simulink model "Assignment_2_3K04"  (R2020a)
settings: Solver=FixedStepAuto  StartTime=0.0  StopTime=1  FixedStep=1e-3  RelTol=1e-3  EnableMultiTasking=on
undefined symbols (not defined in the file): A0, A1, D0, D1, D10, D11, D12, D13, D2, D3, D4, D5, D6, D7, D8, D9, PTA0, PTA1, PTA2, PTB2, PTB23, PTB3, PTB9, PTC16, PTC17, PTC2, PTC3, PTC4, PTD0, PTD1, PTD2, PTD3
libraries: frdmk64flib x20, etargetslib x6, dspstat3 x1
settings Model: ExtModeTrigDuration=5  Creator=Stephen Oh  LastModifiedBy=Ahmed Nazir
settings OptimizationCC: EnhancedBackFolding=on  PassReuseOutputArgsAs=Individual arguments  ZeroExternalMemoryAtStartup=off  ZeroInternalMemoryAtStartup=off  MaxStackSize=64  OptimizeBlockOrder=speed  DifferentSizesBufferReuse=on  OptimizationCustomize=off  EfficientTunableParamExpr=on
settings DebuggingCC: ParameterTunabilityLossMsg=error
settings HardwareCC: ProdBitPerPointer=32  ProdBitPerSizeT=32  ProdBitPerPtrDiffT=32  ProdLargestAtomicInteger=Long  ProdLargestAtomicFloat=Double  ProdWordSize=32  ProdHWDeviceType=ARM Compatible->ARM Cortex
settings SFSimCC: MATLABDynamicMemAlloc=off
settings RTWCC: SystemTargetFile=ert.tlc  HardwareBoard=NXP FRDM-K64F  TemplateMakefile=ert_default_tmf  Toolchain=GNU Tools for ARM Embedded Processors
settings CodeAppCC: ForceParamTrailComments=on  IgnoreCustomStorageClasses=off  OperatorAnnotations=on  SimulinkDataObjDesc=on  SFDataObjDesc=on  InsertBlockDesc=on

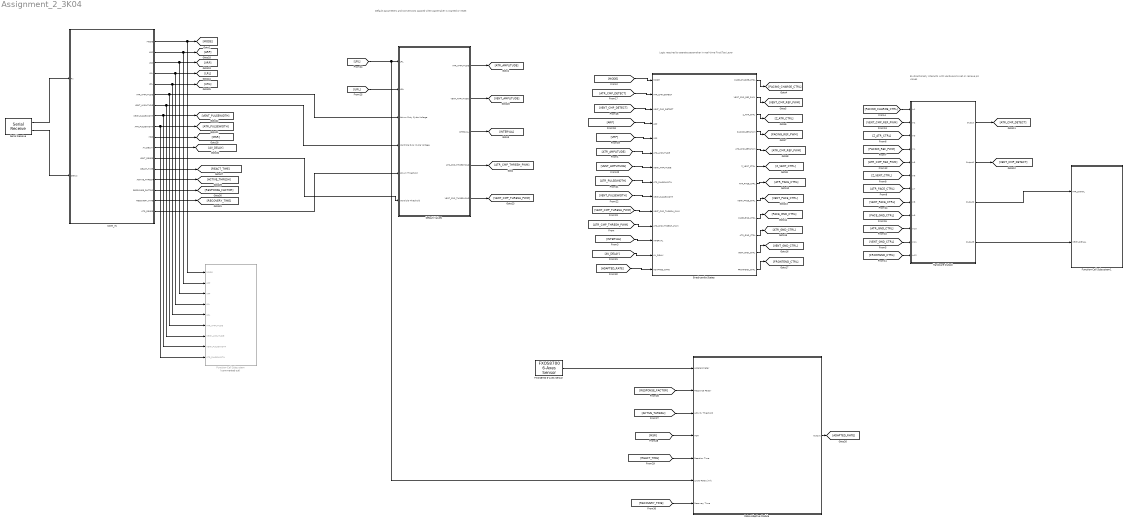
== system Assignment_2_3K04 ==
  note: Default parameters and Conversions passed when
      | pacemaker is started or reset
  note: Logic required to operate pacemaker
      | in real-time
      | First/Top Layer
  note: Bi-directionally interacts with
      | Hardware to set or recieve
      | pin values
  Bradycardia States : Stateflow chart  TreatAsAtomicUnit=on
      settings: PortSchema="{\"entries\":[{\"content\":{\"sides\":[{\"content\":{\"connectorIds\":[\"In2\",\"In3\",\"In4\",\"In5\",\"In6\",\"In7\",\"In8\",\"In9\",\"In10\",\"In11\",\"In12\",\"In1\",\"In13\",\"In14\"]},\"type\":\"ConnectorPlacement.EquallySpacedRectSide\",\"uuid\":\"15e03f69-5c25-4f3e-b3fb-d71978e552f4\"},{\"content\":{\"connectorIds\":[\"Out7\",\"Out12\",\"Out4\",\"Out8\",\"Out10\",\"Out5\",\"Out9\",\"Out3\",\"Out6\",\"Out1\",\"Out2\",\"Out11\"],\"side\":\"RIGHT\"},\"type\":\"ConnectorPlacement.EquallySpacedRectSide\",\"uuid\":\"02171bf1-edb1-4b01-9e56-a8642c556ed6\"},{\"content\":{\"connectorIds\":[],\"side\":\"TOP\"},\"type\":\"ConnectorPlacement.EquallySpacedRectSide\",\"uuid\":\"cc6b5506-3435-4740-9e3f-4dfe15d30bff\"}]},\"type\":\"ConnectorPlacement.EquallySpacedConnector\",\"uuid\":\"0ad55da7-1e65-48d0-a0a4-2620ffa94320\"}],\"packageUris\":[\"http://schema.mathworks.com/mf0/Connector/19700101\"],\"version\":\"1.0\"}"
  COM_IN : Stateflow chart  TreatAsAtomicUnit=on
      settings: PortSchema="{\"entries\":[{\"content\":{\"sides\":[{\"content\":{\"connectorIds\":[\"In1\",\"In2\"]},\"type\":\"ConnectorPlacement.EquallySpacedRectSide\",\"uuid\":\"22fa9edc-2a49-4280-8e8e-0842a45ddb47\"},{\"content\":{\"connectorIds\":[\"Out1\",\"Out2\",\"Out5\",\"Out3\",\"Out4\",\"Out6\",\"Out7\",\"Out8\",\"Out9\",\"Out10\",\"Out11\",\"Out12\",\"Out13\",\"Out14\",\"Out15\",\"Out16\",\"Out17\"],\"side\":\"RIGHT\"},\"type\":\"ConnectorPlacement.EquallySpacedRectSide\",\"uuid\":\"653d204d-01e6-4b1d-8e7b-47ebaddcd032\"},{\"content\":{\"connectorIds\":[],\"side\":\"TOP\"},\"type\":\"ConnectorPlacement.EquallySpacedRectSide\",\"uuid\":\"5fb759fd-937e-492d-8a65-272e5a7048d8\"}]},\"type\":\"ConnectorPlacement.EquallySpacedConnector\",\"uuid\":\"8ef65fa3-58c0-4e1e-983b-59a6af0cca9a\"}],\"packageUris\":[\"http://schema.mathworks.com/mf0/Connector/19700101\"],\"version\":\"1.0\"}"
  Default Values : Subsystem
  FXOS8700 6-Axes Sensor : frdmk64flib/FXOS8700 6-Axes Sensor  Activesensor=Accelerometer only  ODR=800Hz  HybridODR=400Hz  Accelfullrange=-4g to +4g  SampleTime=-1
  Function-Call Subsystem : Subsystem  Commented=on  TreatAsAtomicUnit=on
  Function-Call Subsystem1 : Subsystem  TreatAsAtomicUnit=on
  Hardware Output : Subsystem
  Rate Adaptive Module : Subsystem
  Serial Receive : frdmk64flib/Serial Receive  SCIModule=0  Baudrate=uint32(9600)  Parity=None  StopBits=1  HardwareFlowControl=None  ByteOrder=LittleEndian  DataType=uint8  DataLength=37  BlockingMode=off  OutputStatus=on  SampleTime=-1
  wires:
  [INTERVAL] -> Bradycardia States/1(INTERVAL)
  [ATR_GND_CTRL] -> Hardware Output/10(In10)
  [PACING_REF_PWM] -> Hardware Output/4(In4)
  [Z_VENT_CTRL] -> Hardware Output/6(In6)
  [ATR_PACE_CTRL] -> Hardware Output/7(In7)
  Hardware Output/2(Output1) -> [VENT_CMP_DETECT]
  [PACE_GND_CTRL] -> Hardware Output/9(In9)
  [FRONTEND_CTRL] -> Hardware Output/12(In12)
  [VENT_GND_CTRL] -> Hardware Output/11(In11)
  [Z_ATR_CTRL] -> Hardware Output/3(In3)
  [VENT_PACE_CTRL] -> Hardware Output/8(In8)
  [ATR_CMP_REF_PWM] -> Hardware Output/5(In5)
  [VENT_CMP_REF_PWM] -> Hardware Output/2(In2)
  [PACING_CHARGE_CTRL] -> Hardware Output/1(In1)
  Hardware Output/1(Output) -> [ATR_CMP_DETECT]
  [VENT_CMP_DETECT] -> Bradycardia States/4(VENT_CMP_DETECT)
  [ARP] -> Bradycardia States/5(ARP)
  [VRP] -> Bradycardia States/6(VRP)
  [ATR_CMP_DETECT] -> Bradycardia States/3(ATR_CMP_DETECT)
  [ATR_AMPLITUDE] -> Bradycardia States/7(ATR_AMPLITUDE)
  [VENT_AMPLITUDE] -> Bradycardia States/8(VENT_AMPLITUDE)
  [ATR_PULSEWIDTH] -> Bradycardia States/9(ATR_PULSEWIDTH)
  [VENT_PULSEWIDTH] -> Bradycardia States/10(VENT_PULSEWIDTH)
  Default Values/1(ATR_AMPLITUDE) -> [ATR_AMPLITUDE]
  Default Values/3(INTERVAL) -> [INTERVAL]
  Bradycardia States/3(VENT_PACE_CTRL) -> [VENT_PACE_CTRL]
  Bradycardia States/9(ATR_PACE_CTRL) -> [ATR_PACE_CTRL]
  Bradycardia States/7(PACE_CHARGE_CTRL) -> [PACING_CHARGE_CTRL]
  Bradycardia States/12(VENT_CMP_REF_PWM) -> [VENT_CMP_REF_PWM]
  Bradycardia States/4(Z_ATR_CTRL) -> [Z_ATR_CTRL]
  Bradycardia States/8(PACING_REF_PWM) -> [PACING_REF_PWM]
  Bradycardia States/10(ATR_CMP_REF_PWM) -> [ATR_CMP_REF_PWM]
  Bradycardia States/5(Z_VENT_CTRL) -> [Z_VENT_CTRL]
  Bradycardia States/6(PACE_GND_CTRL) -> [PACE_GND_CTRL]
  Bradycardia States/1(ATR_GND_CTRL) -> [ATR_GND_CTRL]
  Bradycardia States/2(VENT_GND_CTRL) -> [VENT_GND_CTRL]
  Bradycardia States/11(FRONTEND_CTRL) -> [FRONTEND_CTRL]
  [ATR_CMP_THRESH_PWM] -> Bradycardia States/12(ATR_CMP_THRESH_PWM)
  [VENT_CMP_THRESH_PWM] -> Bradycardia States/11(VENT_CMP_THRESH_PWM)
  Serial Receive/1 -> COM_IN/1(Rx)
  Serial Receive/2 -> COM_IN/2(Status)
  COM_IN/1(MODE) -> Function-Call Subsystem/1(MODE), [MODE]
  [MODE] -> Bradycardia States/2(MODE)
  COM_IN/2(ARP) -> Function-Call Subsystem/2(ARP), [ARP]
  COM_IN/5(VRP) -> Function-Call Subsystem/3(VRP), [VRP]
  COM_IN/6(ATR_AMPLITUDE) -> Function-Call Subsystem/6(ATR_AMPLITUDE), Default Values/3(Atrium Duty Cycle Voltage)
  COM_IN/7(VENT_AMPLITUDE) -> Function-Call Subsystem/7(VENT_AMPLITUDE), Default Values/4(Ventricle Duty Cycle Voltage)
  Default Values/2(VENT_AMPLITUDE) -> [VENT_AMPLITUDE]
  COM_IN/3(LRL) -> Function-Call Subsystem/4(LRL), [LRL]
  COM_IN/4(URL) -> Function-Call Subsystem/5(URL), [URL]
  [URL] -> Default Values/2(URL)
  COM_IN/13(REACT_TIME) -> [REACT_TIME]
  COM_IN/10(MSR) -> [MSR]
  COM_IN/14(ACTIVE_THRESH) -> [ACTIVE_THRESH]
  COM_IN/15(RESPONSE_FACTOR) -> [RESPONSE_FACTOR]
  COM_IN/16(RECOVERY_TIME) -> [RECOVERY_TIME]
  COM_IN/11(AV_DELAY) -> [AV_DELAY]
  [AV_DELAY] -> Bradycardia States/13(AV_DELAY)
  [ADAPTED_RATE] -> Bradycardia States/14(ADAPTED_RATE)
  COM_IN/8(VENT_PULSEWIDTH) -> Function-Call Subsystem/8(VENT_PULSEWIDTH), [VENT_PULSEWIDTH]
  COM_IN/9(ATR_PULSEWIDTH) -> Function-Call Subsystem/9(ATR_PULSEWIDTH), [ATR_PULSEWIDTH]
  Default Values/4(ATR_CMP_THRESHOLD) -> [ATR_CMP_THRESH_PWM]
  Default Values/5(VENT_CMP_THRESHOLD) -> [VENT_CMP_THRESH_PWM]
  COM_IN/12(VENT_SENSE) -> Default Values/6(Ventricle Threshold)
  COM_IN/17(ATR_SENSE) -> Default Values/5(Atrium Threshold)
  FXOS8700 6-Axes Sensor/1 -> Rate Adaptive Module/1(Accelerometer)
  Rate Adaptive Module/1(Output) -> [ADAPTED_RATE]
  [RESPONSE_FACTOR] -> Rate Adaptive Module/2(Response Factor)
  [ACTIVE_THRESH] -> Rate Adaptive Module/3(Activity Threshold)
  [MSR] -> Rate Adaptive Module/4(MSR)
  [REACT_TIME] -> Rate Adaptive Module/5(Reaction Time)
  [LRL] -> Rate Adaptive Module/6(Lower Rate Limit), Default Values/1(LRL)
  [RECOVERY_TIME] -> Rate Adaptive Module/7(Recovery Time)
  Hardware Output/3(Output2) -> Function-Call Subsystem1/1(ATR_SIGNAL)
  Hardware Output/4(Output3) -> Function-Call Subsystem1/2(VENT_SIGNAL)

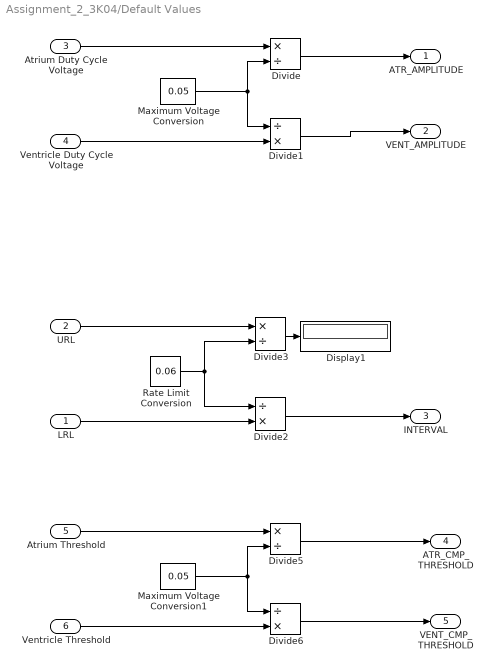
== system Assignment_2_3K04/Default Values ==
  LRL : Inport
  URL : Inport  Port=2
  Atrium Duty Cycle Voltage : Inport  Port=3  OutDataTypeStr=single
  Ventricle Duty Cycle Voltage : Inport  Port=4  OutDataTypeStr=single
  Atrium Threshold : Inport  Port=5  OutDataTypeStr=single
  Ventricle Threshold : Inport  Port=6  OutDataTypeStr=single
  Display1 : Display
  Divide : Product  Inputs=*/  OutDataTypeStr=uint8
  Divide1 : Product  Inputs=/*  OutDataTypeStr=uint8
  Divide2 : Product  Inputs=/*
  Divide3 : Product  Inputs=*/
  Divide5 : Product  Inputs=*/  OutDataTypeStr=uint8
  Divide6 : Product  Inputs=/*  OutDataTypeStr=uint8
  Maximum Voltage Conversion : Constant  Value=0.05
  Maximum Voltage Conversion1 : Constant  Value=0.05
  Rate Limit Conversion : Constant  Value=0.06
  ATR_AMPLITUDE : Outport  OutDataTypeStr=uint8
  VENT_AMPLITUDE : Outport  Port=2  OutDataTypeStr=uint8
  INTERVAL : Outport  Port=3
  ATR_CMP_THRESHOLD : Outport  Port=4  OutDataTypeStr=uint8
  VENT_CMP_THRESHOLD : Outport  Port=5  OutDataTypeStr=uint8
  wires:
  Divide2/1 -> INTERVAL/1
  Maximum Voltage Conversion/1 -> Divide1/1, Divide/2
  Rate Limit Conversion/1 -> Divide3/2, Divide2/1
  URL/1 -> Divide3/1
  Divide3/1 -> Display1/1
  Atrium Duty Cycle Voltage/1 -> Divide/1
  Ventricle Duty Cycle Voltage/1 -> Divide1/2
  Divide/1 -> ATR_AMPLITUDE/1
  Divide1/1 -> VENT_AMPLITUDE/1
  Divide6/1 -> VENT_CMP_THRESHOLD/1
  Maximum Voltage Conversion1/1 -> Divide6/1, Divide5/2
  Atrium Threshold/1 -> Divide5/1
  Divide5/1 -> ATR_CMP_THRESHOLD/1
  Ventricle Threshold/1 -> Divide6/2
  LRL/1 -> Divide2/2

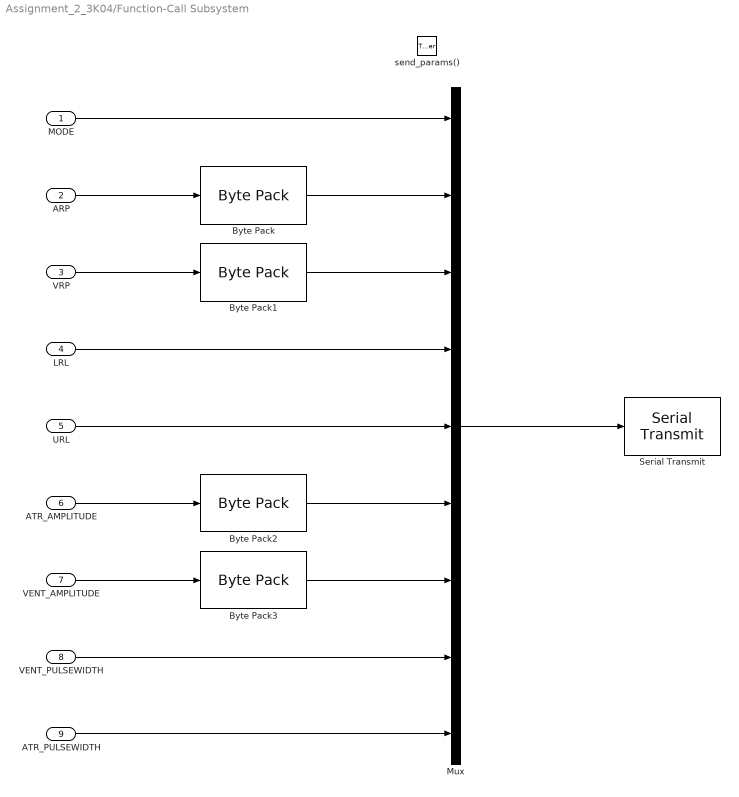
== system Assignment_2_3K04/Function-Call Subsystem ==
  MODE : Inport  OutDataTypeStr=uint8
  ARP : Inport  Port=2
  VRP : Inport  Port=3
  LRL : Inport  Port=4
  URL : Inport  Port=5
  ATR_AMPLITUDE : Inport  Port=6
  VENT_AMPLITUDE : Inport  Port=7
  VENT_PULSEWIDTH : Inport  Port=8
  ATR_PULSEWIDTH : Inport  Port=9
  send_params() : TriggerPort  TriggerType=function-call  IsSimulinkFunction=on  FunctionName=send_params  VariantControl=Variant
  Byte Pack : etargetslib/Byte Pack  datatypes={'uint16'}  byteAlign=1
  Byte Pack1 : etargetslib/Byte Pack  datatypes={'uint16'}  byteAlign=1
  Byte Pack2 : etargetslib/Byte Pack  datatypes={'single'}  byteAlign=1
  Byte Pack3 : etargetslib/Byte Pack  datatypes={'single'}  byteAlign=1
  Mux : Mux  Inputs=9
  Serial Transmit : frdmk64flib/Serial Transmit  SCIModule=0  Baudrate=uint32(9600)  Parity=None  StopBits=1  HardwareFlowControl=None  ByteOrder=LittleEndian  BlockingMode=on  OutputStatus=off
  wires:
  Mux/1 -> Serial Transmit/1
  ARP/1 -> Byte Pack/1
  VRP/1 -> Byte Pack1/1
  LRL/1 -> Mux/4
  URL/1 -> Mux/5
  ATR_AMPLITUDE/1 -> Byte Pack2/1
  VENT_AMPLITUDE/1 -> Byte Pack3/1
  VENT_PULSEWIDTH/1 -> Mux/8
  ATR_PULSEWIDTH/1 -> Mux/9
  MODE/1 -> Mux/1
  Byte Pack/1 -> Mux/2
  Byte Pack1/1 -> Mux/3
  Byte Pack2/1 -> Mux/6
  Byte Pack3/1 -> Mux/7

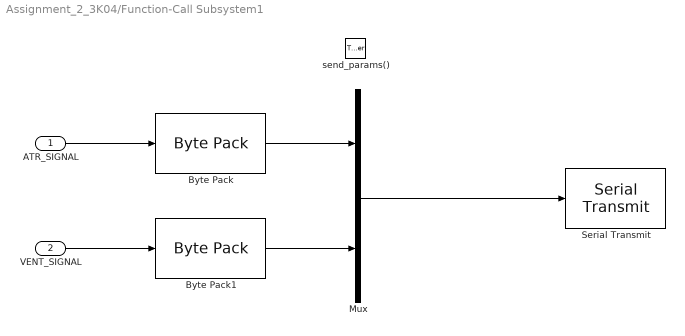
== system Assignment_2_3K04/Function-Call Subsystem1 ==
  ATR_SIGNAL : Inport  OutDataTypeStr=double
  VENT_SIGNAL : Inport  Port=2  OutDataTypeStr=double
  send_params() : TriggerPort  TriggerType=function-call  IsSimulinkFunction=on  FunctionName=send_params  VariantControl=Variant
  Byte Pack : etargetslib/Byte Pack  datatypes={'double'}  byteAlign=1
  Byte Pack1 : etargetslib/Byte Pack  datatypes={'double'}  byteAlign=1
  Mux : Mux  Inputs=2
  Serial Transmit : frdmk64flib/Serial Transmit  SCIModule=0  Baudrate=uint32(9600)  Parity=None  StopBits=1  HardwareFlowControl=None  ByteOrder=LittleEndian  BlockingMode=on  OutputStatus=off
  wires:
  ATR_SIGNAL/1 -> Byte Pack/1
  Mux/1 -> Serial Transmit/1
  VENT_SIGNAL/1 -> Byte Pack1/1
  Byte Pack/1 -> Mux/1
  Byte Pack1/1 -> Mux/2

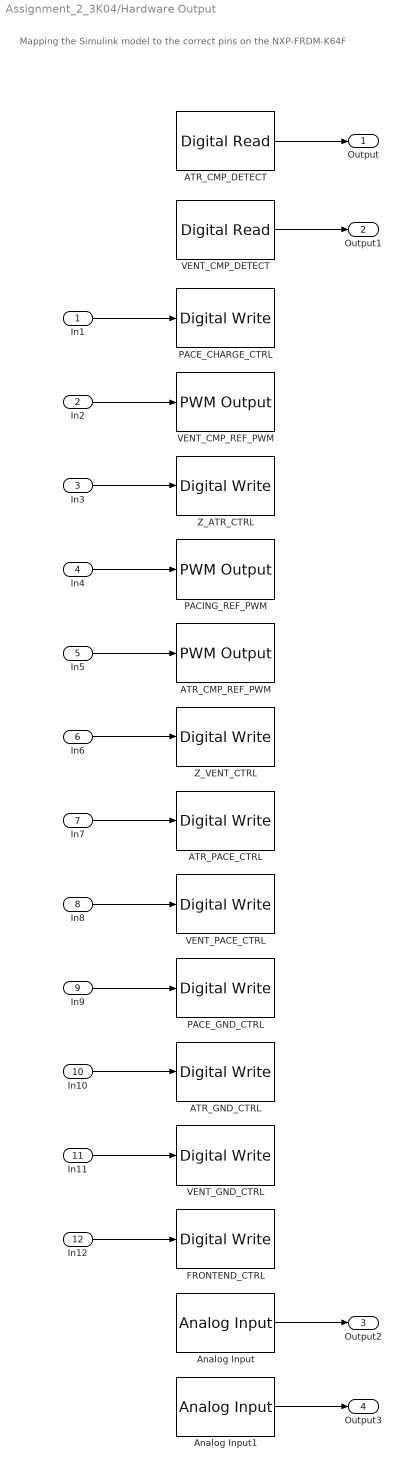
== system Assignment_2_3K04/Hardware Output ==
  note: Mapping the Simulink model to the correct pins
      | on the NXP-FRDM-K64F
  In1 : Inport
  In2 : Inport  Port=2
  In3 : Inport  Port=3
  In4 : Inport  Port=4
  In5 : Inport  Port=5
  In6 : Inport  Port=6
  In7 : Inport  Port=7
  In8 : Inport  Port=8
  In9 : Inport  Port=9
  In10 : Inport  Port=10
  In11 : Inport  Port=11
  In12 : Inport  Port=12
  ATR_CMP_DETECT : frdmk64flib/Digital Read  Whichpin=PTC16 (D0)  SampleTime=-1
  ATR_CMP_REF_PWM : frdmk64flib/PWM Output  Whichpin=PTC2 (D6)  InitialFrequency=2000  InitialDutyCycle=30
  ATR_GND_CTRL : frdmk64flib/Digital Write  Whichpin=PTD2 (D11)
  ATR_PACE_CTRL : frdmk64flib/Digital Write  Whichpin=PTA0 (D8)
  Analog Input : frdmk64flib/Analog Input  Whichpin=PTB2 (A0)  SampleTime=-1
  Analog Input1 : frdmk64flib/Analog Input  Whichpin=PTB3 (A1)  SampleTime=-1
  FRONTEND_CTRL : frdmk64flib/Digital Write  Whichpin=PTD1 (D13)
  PACE_CHARGE_CTRL : frdmk64flib/Digital Write  Whichpin=PTB9 (D2)
  PACE_GND_CTRL : frdmk64flib/Digital Write  Whichpin=PTD0 (D10)
  PACING_REF_PWM : frdmk64flib/PWM Output  Whichpin=PTA2 (D5)  InitialFrequency=2000  InitialDutyCycle=30
  VENT_CMP_DETECT : frdmk64flib/Digital Read  Whichpin=PTC17 (D1)  SampleTime=-1
  VENT_CMP_REF_PWM : frdmk64flib/PWM Output  Whichpin=PTA1 (D3)  InitialFrequency=2000  InitialDutyCycle=30
  VENT_GND_CTRL : frdmk64flib/Digital Write  Whichpin=PTD3 (D12)
  VENT_PACE_CTRL : frdmk64flib/Digital Write  Whichpin=PTC4 (D9)
  Z_ATR_CTRL : frdmk64flib/Digital Write  Whichpin=PTB23 (D4)
  Z_VENT_CTRL : frdmk64flib/Digital Write  Whichpin=PTC3 (D7)
  Output : Outport
  Output1 : Outport  Port=2
  Output2 : Outport  Port=3  OutDataTypeStr=double
  Output3 : Outport  Port=4  OutDataTypeStr=double
  wires:
  In1/1 -> PACE_CHARGE_CTRL/1
  ATR_CMP_DETECT/1 -> Output/1
  VENT_CMP_DETECT/1 -> Output1/1
  In2/1 -> VENT_CMP_REF_PWM/1
  In3/1 -> Z_ATR_CTRL/1
  In4/1 -> PACING_REF_PWM/1
  In5/1 -> ATR_CMP_REF_PWM/1
  In6/1 -> Z_VENT_CTRL/1
  In7/1 -> ATR_PACE_CTRL/1
  In8/1 -> VENT_PACE_CTRL/1
  In9/1 -> PACE_GND_CTRL/1
  In10/1 -> ATR_GND_CTRL/1
  In11/1 -> VENT_GND_CTRL/1
  In12/1 -> FRONTEND_CTRL/1
  Analog Input/1 -> Output2/1
  Analog Input1/1 -> Output3/1

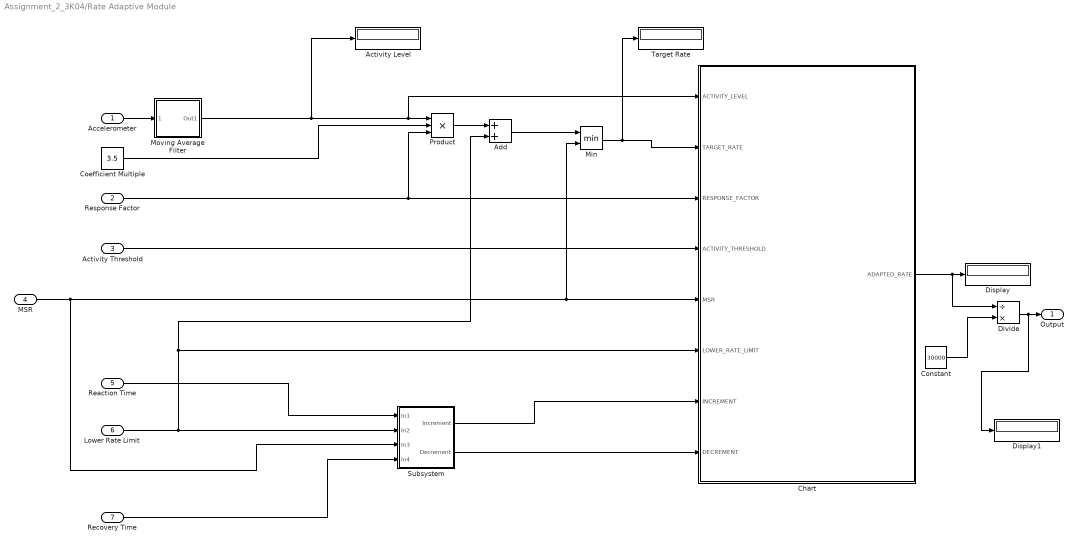
== system Assignment_2_3K04/Rate Adaptive Module ==
  Accelerometer : Inport
  Response Factor : Inport  Port=2
  Activity Threshold : Inport  Port=3
  MSR : Inport  Port=4
  Reaction Time : Inport  Port=5
  Lower Rate Limit : Inport  Port=6
  Recovery Time : Inport  Port=7
  Activity Level : Display
  Add : Sum
  Chart : Stateflow chart  TreatAsAtomicUnit=on
      settings: PortSchema="{\"entries\":[{\"content\":{\"sides\":[{\"content\":{\"connectorIds\":[\"In1\",\"In3\",\"In2\",\"In6\",\"In8\",\"In7\",\"In4\",\"In5\"]},\"type\":\"ConnectorPlacement.EquallySpacedRectSide\",\"uuid\":\"efebee7e-2c09-4b25-ba04-904f72c011ed\"},{\"content\":{\"connectorIds\":[\"Out1\"],\"side\":\"RIGHT\"},\"type\":\"ConnectorPlacement.EquallySpacedRectSide\",\"uuid\":\"6322cc63-1b7a-423a-b49b-7b27e71e0c32\"},{\"content\":{\"connectorIds\":[],\"side\":\"TOP\"},\"type\":\"ConnectorPlacement.EquallySpacedRectSide\",\"uuid\":\"daf2dbd4-7676-46e9-bb01-958bd0e2e14e\"}]},\"type\":\"ConnectorPlacement.EquallySpacedConnector\",\"uuid\":\"43c3c7b3-b94c-45f5-b310-1a430cfb2b71\"}],\"packageUris\":[\"http://schema.mathworks.com/mf0/Connector/19700101\"],\"version\":\"1.0\"}"
  Coefficient Multiple : Constant  Value=3.5
  Constant : Constant  Value=30000
  Display : Display
  Display1 : Display
  Divide : Product  Inputs=/*
  Min : MinMax  Inputs=2
  Moving Average Filter : Subsystem
  Product : Product  Inputs=3
  Subsystem : Subsystem
  Target Rate : Display
  Output : Outport
  wires:
  Recovery Time/1 -> Subsystem/4(In4)
  MSR/1 -> Subsystem/3(In3), Min/2, Chart/8(MSR)
  Subsystem/1(Increment) -> Chart/4(INCREMENT)
  Activity Threshold/1 -> Chart/6(ACTIVITY_THRESHOLD)
  Response Factor/1 -> Product/3, Chart/2(RESPONSE_FACTOR)
  Lower Rate Limit/1 -> Subsystem/2(In2), Chart/7(LOWER_RATE_LIMIT), Add/2
  Add/1 -> Min/1
  Product/1 -> Add/1
  Min/1 -> Target Rate/1, Chart/3(TARGET_RATE)
  Reaction Time/1 -> Subsystem/1(In1)
  Subsystem/2(Decrement) -> Chart/5(DECREMENT)
  Chart/1(ADAPTED_RATE) -> Divide/1, Display/1
  Coefficient Multiple/1 -> Product/2
  Divide/1 -> Display1/1, Output/1
  Constant/1 -> Divide/2
  Moving Average Filter/1(Out1) -> Activity Level/1, Chart/1(ACTIVITY_LEVEL), Product/1
  Accelerometer/1 -> Moving Average Filter/1(Accelerometer)

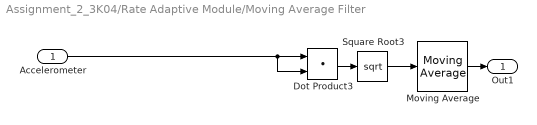
== system Assignment_2_3K04/Rate Adaptive Module/Moving Average Filter ==
  Accelerometer : Inport
  Dot Product3 : DotProduct  InputSameDT=on  OutDataTypeStr=Inherit: Inherit via internal rule
  Moving Average : dspstat3/Moving Average  Method=Sliding window  ForgettingFactorPort=off  SpecifyWindowLength=on  WindowLength=500  ForgettingFactor=0.9  SimulateUsing=Code generation
  Square Root3 : Sqrt  SaturateOnIntegerOverflow=on
  Out1 : Outport
  wires:
  Accelerometer/1 -> Dot Product3/2, Dot Product3/1
  Dot Product3/1 -> Square Root3/1
  Square Root3/1 -> Moving Average/1
  Moving Average/1 -> Out1/1

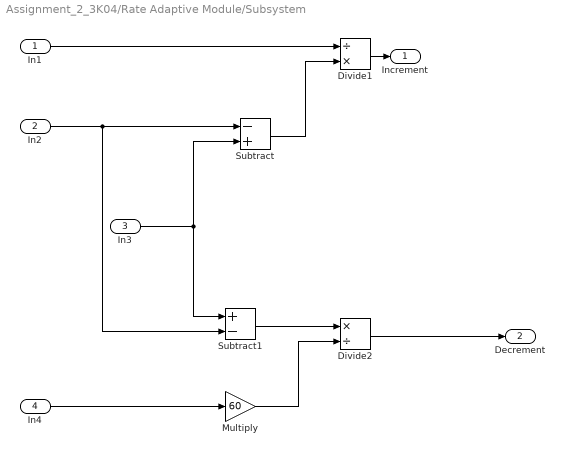
== system Assignment_2_3K04/Rate Adaptive Module/Subsystem ==
  In1 : Inport
  In2 : Inport  Port=2
  In3 : Inport  Port=3
  In4 : Inport  Port=4
  Divide1 : Product  Inputs=/*  OutDataTypeStr=uint8  RndMeth=Ceiling
  Divide2 : Product  Inputs=*/  OutDataTypeStr=uint8  RndMeth=Ceiling  SaturateOnIntegerOverflow=on
  Multiply : Gain  Gain=60
  Subtract : Sum  Inputs=-+
  Subtract1 : Sum  Inputs=+-
  Increment : Outport
  Decrement : Outport  Port=2
  wires:
  Multiply/1 -> Divide2/2
  In2/1 -> Subtract1/2, Subtract/1
  In3/1 -> Subtract/2, Subtract1/1
  Divide1/1 -> Increment/1
  In1/1 -> Divide1/1
  Subtract1/1 -> Divide2/1
  Subtract/1 -> Divide1/2
  In4/1 -> Multiply/1
  Divide2/1 -> Decrement/1

== stateflow chart Assignment_2_3K04/COM_IN ==
  state SET_PARAM
    entry:
    MODE = Rx(3);
    LRL = Rx(4);
    URL = Rx(5);
    ATR_AMPLITUDE = typecast(Rx(6:9),'single');
    VENT_AMPLITUDE = typecast(Rx(10:13),'single');
    ATR_PULSEWIDTH = Rx(14);
    VENT_PULSEWIDTH = Rx(15);
    ARP = typecast(Rx(16:17),'uint16');
    VRP = typecast(Rx(18:19),'uint16');
    ATR_SENSE = typecast(Rx(20:23),'single');
    VENT_SENSE = typecast(Rx(24:27),'single');
    MSR = Rx(28);
    RECOVERY_TIME = Rx(29);
    REACT_TIME = Rx(30);
    RESPONSE_FACTOR = Rx(31);
    ACTIVE_THRESH = typecast(Rx(32:35),'single');
    AV_DELAY = typecast(Rx(36:37),'uint16');
    %Get the values from DCM
  state INITIAL
    %Set all Nomial Values
    entry:
    MODE = 5;
    LRL = 60;
    URL = 120;
    ATR_AMPLITUDE = 5;
    VENT_AMPLITUDE = 5;
    ATR_PULSEWIDTH = 2;
    VENT_PULSEWIDTH = 2;
    ARP = 250;
    VRP = 250;
    ATR_SENSE = 4;
    VENT_SENSE = 4;
    MSR = 100;
    RECOVERY_TIME = 2;
    REACT_TIME = 10;
    RESPONSE_FACTOR = 16;
    ACTIVE_THRESH = 1.1;
    AV_DELAY = 100;
  state STANDBY
    %Wait for COM Data
  state ECHO_PARAM
    entry:
    send_params()
  state INITIAL1 [commented out]
    %Set all Nomial Values
    entry:
    MODE = 0;
    LRL = 60;
    URL = 120;
    ATR_AMPLITUDE = 5;
    VENT_AMPLITUDE = 5;
    ATR_PULSEWIDTH = 1;
    VENT_PULSEWIDTH = 1;
    ARP = 250;
    VRP = 320;
    ATR_SENSE = 4;
    VENT_SENSE = 4;
    MSR = 120;
    RECOVERY_TIME = 5;
    REACT_TIME = 30;
    RESPONSE_FACTOR = 8;
    ACTIVE_THRESH = 0;
    AV_DELAY = 150;
  (default) -> INITIAL
  SET_PARAM -> STANDBY
  (junction 13) -> SET_PARAM [order 1] : [Rx(2) == hex2dec('55')]
  (junction 12) -> STANDBY [order 2]
  INITIAL -> STANDBY
  STANDBY -> (junction 12) : [Status==0]
  (junction 12) -> (junction 13) [order 1] : [Rx(1) == hex2dec('16')]
  (junction 13) -> ECHO_PARAM [order 2] : [Rx(2) == hex2dec('22')]
  ECHO_PARAM -> STANDBY
  data: Rx input uint8; Status input uint8; MODE output uint8; ARP output uint16; LRL output uint8; URL output uint8; VRP output uint16; ATR_AMPLITUDE output single; VENT_AMPLITUDE output single; VENT_PULSEWIDTH output uint8; ATR_PULSEWIDTH output uint8; MSR output uint8; AV_DELAY output uint16; VENT_SENSE output single; REACT_TIME output uint8; ACTIVE_THRESH output single; RESPONSE_FACTOR output uint8; RECOVERY_TIME output uint8; ATR_SENSE output single

== stateflow chart Assignment_2_3K04/Rate Adaptive Module/Chart ==
  state RateSelect
    entry:
    ADAPTED_RATE = LOWER_RATE_LIMIT
  state Increment
    entry:
    ADAPTED_RATE = ADAPTED_RATE + INCREMENT
  state TargetRateAchieved
  state Decrement
    entry:
    ADAPTED_RATE = ADAPTED_RATE - DECREMENT
  Increment -> Increment [order 2] : after(1000, msec) [ACTIVITY_LEVEL > ACTIVITY_THRESHOLD]
  (default) -> RateSelect
  Increment -> TargetRateAchieved [order 1] : [ADAPTED_RATE >= TARGET_RATE ]
  RateSelect -> Increment [order 1] : [ACTIVITY_LEVEL > ACTIVITY_THRESHOLD]
  RateSelect -> RateSelect [order 2] : [ACTIVITY_LEVEL < ACTIVITY_THRESHOLD]
  Decrement -> RateSelect [order 3] : [ADAPTED_RATE <= LOWER_RATE_LIMIT]
  Decrement -> Increment [order 1] : after(1000, msec) [ACTIVITY_LEVEL > ACTIVITY_THRESHOLD]
  Increment -> Decrement [order 3] : after(1000, msec) [ACTIVITY_LEVEL < ACTIVITY_THRESHOLD]
  TargetRateAchieved -> Decrement : [ACTIVITY_LEVEL < ACTIVITY_THRESHOLD]
  Decrement -> Decrement [order 2] : after(1000, msec) [ACTIVITY_LEVEL < ACTIVITY_THRESHOLD]
  data: ACTIVITY_LEVEL input; RESPONSE_FACTOR input; ADAPTED_RATE output; TARGET_RATE input; INCREMENT input; DECREMENT input; ACTIVITY_THRESHOLD input; LOWER_RATE_LIMIT input; MSR input

== stateflow chart Assignment_2_3K04/Bradycardia States ==
  note: Second/Structural Layer
  note: Mode Select with Conditional transition to 4 modes
  state ModeSelect
  state AOO [group]
    state Charging
      entry:
      %
      %Charging capacitor C22
      %
      FRONTEND_CTRL = HIGH
      ATR_PACE_CTRL = LOW
      VENT_PACE_CTRL = LOW
      PACING_REF_PWM = ATR_AMPLITUDE
      PACE_CHARGE_CTRL = HIGH
      %
      %Charge release of capacitor C21 into Atrium ground
      %
      PACE_GND_CTRL = HIGH
      VENT_PACE_CTRL = LOW
      Z_ATR_CTRL = LOW
      Z_VENT_CTRL = LOW
      ATR_PACE_CTRL = LOW
      ATR_GND_CTRL = HIGH
      VENT_GND_CTRL = LOW
    state Discharging
      entry:
      %
      %Charge release of capacitor C22 to charge capacitor C21
      %
      PACE_CHARGE_CTRL = LOW
      PACE_GND_CTRL = HIGH
      VENT_PACE_CTRL = LOW
      VENT_GND_CTRL = LOW
      Z_VENT_CTRL = LOW
      Z_ATR_CTRL = LOW
      ATR_GND_CTRL = LOW
      ATR_PACE_CTRL = HIGH
    AOO.Charging -> AOO.Discharging [order 1] : after(delayINTERVAL, msec)
    AOO.Discharging -> AOO.Charging : after(delayATR_PULSEWIDTH, msec)
  state VOO [group]
    state Charging
      entry:
      %
      %Charging capacitor C22
      %
      FRONTEND_CTRL = HIGH
      ATR_PACE_CTRL = LOW
      VENT_PACE_CTRL = LOW
      PACING_REF_PWM = VENT_AMPLITUDE
      PACE_CHARGE_CTRL = HIGH
      %
      %Charge release of capacitor C21 into Ventricle ground
      %
      PACE_GND_CTRL = HIGH
      VENT_PACE_CTRL = LOW
      Z_ATR_CTRL = LOW
      Z_VENT_CTRL = LOW
      ATR_PACE_CTRL = LOW
      ATR_GND_CTRL = LOW
      VENT_GND_CTRL = HIGH
    state Discharging
      entry:
      %
      %Charge release of capacitor C22 to charge capacitor C21
      %
      PACE_CHARGE_CTRL = LOW
      PACE_GND_CTRL = HIGH
      ATR_PACE_CTRL = LOW
      ATR_GND_CTRL = LOW
      Z_VENT_CTRL = LOW
      Z_ATR_CTRL = LOW
      VENT_GND_CTRL = LOW
      VENT_PACE_CTRL = HIGH
    VOO.Charging -> VOO.Discharging [order 1] : after(delayINTERVAL, msec)
    VOO.Discharging -> VOO.Charging : after(delayVENT_PULSEWIDTH, msec)
  state AAI [group]
    state Transition
      %Check for sense outside atrium refractory period
    state Discharging
      entry:
      %Charge release of capacitor C22 to charge capacitor C21
      %
      PACE_CHARGE_CTRL = LOW
      PACE_GND_CTRL = HIGH
      VENT_PACE_CTRL = LOW
      VENT_GND_CTRL = LOW
      Z_VENT_CTRL = LOW
      Z_ATR_CTRL = LOW
      ATR_GND_CTRL = LOW
      ATR_PACE_CTRL = HIGH
    state Charging
      entry:
      %
      %Turn sensing on
      FRONTEND_CTRL = HIGH
      ATR_CMP_REF_PWM = ATR_CMP_THRESH_PWM
      %Charging capacitor C22
      %
      ATR_PACE_CTRL = LOW
      VENT_PACE_CTRL = LOW
      PACING_REF_PWM = ATR_AMPLITUDE
      PACE_CHARGE_CTRL = HIGH
      %Charge release of capacitor C21 into Atrium ground
      PACE_GND_CTRL = HIGH
      VENT_PACE_CTRL = LOW
      Z_ATR_CTRL = LOW
      Z_VENT_CTRL = LOW
      ATR_PACE_CTRL = LOW
      ATR_GND_CTRL = HIGH
      VENT_GND_CTRL = LOW
    AAI.Transition -> AAI.Discharging [order 1] : after(delayINTERVAL-delayARP, msec)
    AAI.Transition -> AAI.Charging [order 2] : [ATR_CMP_DETECT == HIGH]
    AAI.Charging -> AAI.Transition [order 1] : after(delayARP, msec)
    AAI.Discharging -> AAI.Charging : after(delayATR_PULSEWIDTH, msec)
  state VVI [group]
    state Transition
      %Check for sense outside ventricle refractory period
    state Charging
      entry:
      %
      %Turn sensing on
      FRONTEND_CTRL = HIGH
      VENT_CMP_REF_PWM = VENT_CMP_THRESH_PWM
      %Charging capacitor C22
      %
      ATR_PACE_CTRL = LOW
      VENT_PACE_CTRL = LOW
      PACING_REF_PWM = VENT_AMPLITUDE
      PACE_CHARGE_CTRL = HIGH
      %Charge release of capacitor C21 into Ventricle ground
      PACE_GND_CTRL = HIGH
      VENT_PACE_CTRL = LOW
      Z_ATR_CTRL = LOW
      Z_VENT_CTRL = LOW
      ATR_PACE_CTRL = LOW
      ATR_GND_CTRL = LOW
      VENT_GND_CTRL = HIGH
    state Discharging
      entry:
      %Charge release of capacitor C22 to charge capacitor C21
      %
      PACE_CHARGE_CTRL = LOW
      PACE_GND_CTRL = HIGH
      ATR_PACE_CTRL = LOW
      ATR_GND_CTRL = LOW
      Z_VENT_CTRL = LOW
      Z_ATR_CTRL = LOW
      VENT_GND_CTRL = LOW
      VENT_PACE_CTRL = HIGH
    VVI.Transition -> VVI.Discharging [order 1] : after(delayINTERVAL-delayVRP, msec)
    VVI.Transition -> VVI.Charging [order 2] : [VENT_CMP_DETECT == HIGH]
    VVI.Charging -> VVI.Transition [order 1] : after(delayVRP, msec)
    VVI.Discharging -> VVI.Charging : after(delayVENT_PULSEWIDTH, msec)
  state AOOR [group]
    state Charging
      entry:
      %
      %Charging capacitor C22
      %
      FRONTEND_CTRL = HIGH
      ATR_PACE_CTRL = LOW
      VENT_PACE_CTRL = LOW
      PACING_REF_PWM = ATR_AMPLITUDE
      PACE_CHARGE_CTRL = HIGH
      %
      %Charge release of capacitor C21 into Atrium ground
      %
      PACE_GND_CTRL = HIGH
      VENT_PACE_CTRL = LOW
      Z_ATR_CTRL = LOW
      Z_VENT_CTRL = LOW
      ATR_PACE_CTRL = LOW
      ATR_GND_CTRL = HIGH
      VENT_GND_CTRL = LOW
    state Discharging
      entry:
      %
      %Charge release of capacitor C22 to charge capacitor C21
      %
      PACE_CHARGE_CTRL = LOW
      PACE_GND_CTRL = HIGH
      VENT_PACE_CTRL = LOW
      VENT_GND_CTRL = LOW
      Z_VENT_CTRL = LOW
      Z_ATR_CTRL = LOW
      ATR_GND_CTRL = LOW
      ATR_PACE_CTRL = HIGH
    AOOR.Charging -> AOOR.Discharging [order 1] : after(ADAPTED_RATE, msec)
    AOOR.Discharging -> AOOR.Charging : after(delayATR_PULSEWIDTH, msec)
  state VOOR [group]
    state Charging
      entry:
      %
      %Charging capacitor C22
      %
      FRONTEND_CTRL = HIGH
      ATR_PACE_CTRL = LOW
      VENT_PACE_CTRL = LOW
      PACING_REF_PWM = VENT_AMPLITUDE
      PACE_CHARGE_CTRL = HIGH
      %
      %Charge release of capacitor C21 into Ventricle ground
      %
      PACE_GND_CTRL = HIGH
      VENT_PACE_CTRL = LOW
      Z_ATR_CTRL = LOW
      Z_VENT_CTRL = LOW
      ATR_PACE_CTRL = LOW
      ATR_GND_CTRL = LOW
      VENT_GND_CTRL = HIGH
    state Discharging
      entry:
      %
      %Charge release of capacitor C22 to charge capacitor C21
      %
      PACE_CHARGE_CTRL = LOW
      PACE_GND_CTRL = HIGH
      ATR_PACE_CTRL = LOW
      ATR_GND_CTRL = LOW
      Z_VENT_CTRL = LOW
      Z_ATR_CTRL = LOW
      VENT_GND_CTRL = LOW
      VENT_PACE_CTRL = HIGH
    VOOR.Charging -> VOOR.Discharging [order 1] : after(ADAPTED_RATE, msec)
    VOOR.Discharging -> VOOR.Charging : after(delayVENT_PULSEWIDTH, msec)
  state AAIR [group]
    state Transition
      %Check for sense outside atrium refractory period
    state Discharging
      entry:
      %Charge release of capacitor C22 to charge capacitor C21
      %
      PACE_CHARGE_CTRL = LOW
      PACE_GND_CTRL = HIGH
      VENT_PACE_CTRL = LOW
      VENT_GND_CTRL = LOW
      Z_VENT_CTRL = LOW
      Z_ATR_CTRL = LOW
      ATR_GND_CTRL = LOW
      ATR_PACE_CTRL = HIGH
    state Charging
      entry:
      %
      %Turn sensing on
      FRONTEND_CTRL = HIGH
      ATR_CMP_REF_PWM = ATR_CMP_THRESH_PWM
      %Charging capacitor C22
      %
      ATR_PACE_CTRL = LOW
      VENT_PACE_CTRL = LOW
      PACING_REF_PWM = ATR_AMPLITUDE
      PACE_CHARGE_CTRL = HIGH
      %Charge release of capacitor C21 into Atrium ground
      PACE_GND_CTRL = HIGH
      VENT_PACE_CTRL = LOW
      Z_ATR_CTRL = LOW
      Z_VENT_CTRL = LOW
      ATR_PACE_CTRL = LOW
      ATR_GND_CTRL = HIGH
      VENT_GND_CTRL = LOW
    AAIR.Transition -> AAIR.Discharging [order 1] : after(ADAPTED_RATE - delayARP, msec)
    AAIR.Transition -> AAIR.Charging [order 2] : [ATR_CMP_DETECT == HIGH]
    AAIR.Charging -> AAIR.Transition [order 1] : after(delayARP, msec)
    AAIR.Discharging -> AAIR.Charging : after(delayATR_PULSEWIDTH, msec)
  state VVIR [group]
    state Transition
      %Check for sense outside ventricle refractory period
    state Charging
      entry:
      %
      %Turn sensing on
      FRONTEND_CTRL = HIGH
      VENT_CMP_REF_PWM = VENT_CMP_THRESH_PWM
      %Charging capacitor C22
      %
      ATR_PACE_CTRL = LOW
      VENT_PACE_CTRL = LOW
      PACING_REF_PWM = VENT_AMPLITUDE
      PACE_CHARGE_CTRL = HIGH
      %Charge release of capacitor C21 into Ventricle ground
      PACE_GND_CTRL = HIGH
      VENT_PACE_CTRL = LOW
      Z_ATR_CTRL = LOW
      Z_VENT_CTRL = LOW
      ATR_PACE_CTRL = LOW
      ATR_GND_CTRL = LOW
      VENT_GND_CTRL = HIGH
    state Discharging
      entry:
      %Charge release of capacitor C22 to charge capacitor C21
      %
      PACE_CHARGE_CTRL = LOW
      PACE_GND_CTRL = HIGH
      ATR_PACE_CTRL = LOW
      ATR_GND_CTRL = LOW
      Z_VENT_CTRL = LOW
      Z_ATR_CTRL = LOW
      VENT_GND_CTRL = LOW
      VENT_PACE_CTRL = HIGH
    VVIR.Transition -> VVIR.Discharging [order 1] : after(ADAPTED_RATE-delayVRP, msec)
    VVIR.Transition -> VVIR.Charging [order 2] : [VENT_CMP_DETECT == HIGH]
    VVIR.Charging -> VVIR.Transition [order 1] : after(delayVRP, msec)
    VVIR.Discharging -> VVIR.Charging : after(delayVENT_PULSEWIDTH, msec)
  state DOO [group]
    state Discharging_to_Atrium
      entry:
      %
      %Charge release of capacitor C22 to charge capacitor C21
      %
      PACE_CHARGE_CTRL = LOW
      PACE_GND_CTRL = HIGH
      VENT_PACE_CTRL = LOW
      VENT_GND_CTRL = LOW
      Z_VENT_CTRL = LOW
      Z_ATR_CTRL = LOW
      ATR_GND_CTRL = LOW
      ATR_PACE_CTRL = HIGH
    state Charging_for_Atrium
      entry:
      %
      %Charging capacitor C22
      %
      FRONTEND_CTRL = HIGH
      ATR_PACE_CTRL = LOW
      VENT_PACE_CTRL = LOW
      PACING_REF_PWM = ATR_AMPLITUDE
      PACE_CHARGE_CTRL = HIGH
      %
      %Charge release of capacitor C21 into Atrium ground
      %
      PACE_GND_CTRL = HIGH
      VENT_PACE_CTRL = LOW
      Z_ATR_CTRL = LOW
      Z_VENT_CTRL = LOW
      ATR_PACE_CTRL = LOW
      ATR_GND_CTRL = HIGH
      VENT_GND_CTRL = LOW
    note: NOTE:
        | -AV_DELAY does not occur after ATR_PULSEWIDTH
        | -AV_DELAY starts at the same time as ATR_PULSEWIDTH
        | -ATR_PURLSEWIDTH transition still required for pace width
    state Charging
      entry:
      %
      %Charging capacitor C22
      %
      ATR_PACE_CTRL = LOW
      VENT_PACE_CTRL = LOW
      PACING_REF_PWM = VENT_AMPLITUDE
      PACE_CHARGE_CTRL = HIGH
      %
      %Charge release of capacitor C21 into Ventricle ground
      %
      PACE_GND_CTRL = HIGH
      VENT_PACE_CTRL = LOW
      Z_ATR_CTRL = LOW
      Z_VENT_CTRL = LOW
      ATR_PACE_CTRL = LOW
      ATR_GND_CTRL = LOW
      VENT_GND_CTRL = HIGH
    state Discharging
      entry:
      %
      %Charge release of capacitor C22 to charge capacitor C21
      %
      PACE_CHARGE_CTRL = LOW
      PACE_GND_CTRL = HIGH
      ATR_PACE_CTRL = LOW
      ATR_GND_CTRL = LOW
      Z_VENT_CTRL = LOW
      Z_ATR_CTRL = LOW
      VENT_GND_CTRL = LOW
      VENT_PACE_CTRL = HIGH
    DOO.Charging_for_Atrium -> DOO.Discharging_to_Atrium [order 1] : after(delayINTERVAL-delayAV_DELAY, msec)
    DOO.Discharging -> DOO.Charging_for_Atrium : after(delayVENT_PULSEWIDTH, msec)
    DOO.Discharging_to_Atrium -> DOO.Charging : after(delayATR_PULSEWIDTH, msec)
    DOO.Charging -> DOO.Discharging : after(delayAV_DELAY, msec)
  state DOOR [group]
    state Discharging_to_Atrium
      entry:
      %
      %Charge release of capacitor C22 to charge capacitor C21
      %
      PACE_CHARGE_CTRL = LOW
      PACE_GND_CTRL = HIGH
      VENT_PACE_CTRL = LOW
      VENT_GND_CTRL = LOW
      Z_VENT_CTRL = LOW
      Z_ATR_CTRL = LOW
      ATR_GND_CTRL = LOW
      ATR_PACE_CTRL = HIGH
    state Charging_for_Atrium
      entry:
      %
      %Charging capacitor C22
      %
      FRONTEND_CTRL = HIGH
      ATR_PACE_CTRL = LOW
      VENT_PACE_CTRL = LOW
      PACING_REF_PWM = ATR_AMPLITUDE
      PACE_CHARGE_CTRL = HIGH
      %
      %Charge release of capacitor C21 into Atrium ground
      %
      PACE_GND_CTRL = HIGH
      VENT_PACE_CTRL = LOW
      Z_ATR_CTRL = LOW
      Z_VENT_CTRL = LOW
      ATR_PACE_CTRL = LOW
      ATR_GND_CTRL = HIGH
      VENT_GND_CTRL = LOW
    note: NOTE:
        | -AV_DELAY does not occur after ATR_PULSEWIDTH
        | -AV_DELAY starts at the same time as ATR_PULSEWIDTH
        | -ATR_PURLSEWIDTH transition still required for pace width
    state Charging
      entry:
      %
      %Charging capacitor C22
      %
      ATR_PACE_CTRL = LOW
      VENT_PACE_CTRL = LOW
      PACING_REF_PWM = VENT_AMPLITUDE
      PACE_CHARGE_CTRL = HIGH
      %
      %Charge release of capacitor C21 into Ventricle ground
      %
      PACE_GND_CTRL = HIGH
      VENT_PACE_CTRL = LOW
      Z_ATR_CTRL = LOW
      Z_VENT_CTRL = LOW
      ATR_PACE_CTRL = LOW
      ATR_GND_CTRL = LOW
      VENT_GND_CTRL = HIGH
    state Discharging
      entry:
      %
      %Charge release of capacitor C22 to charge capacitor C21
      %
      PACE_CHARGE_CTRL = LOW
      PACE_GND_CTRL = HIGH
      ATR_PACE_CTRL = LOW
      ATR_GND_CTRL = LOW
      Z_VENT_CTRL = LOW
      Z_ATR_CTRL = LOW
      VENT_GND_CTRL = LOW
      VENT_PACE_CTRL = HIGH
    DOOR.Charging_for_Atrium -> DOOR.Discharging_to_Atrium [order 1] : after(ADAPTED_RATE-delayAV_DELAY, msec)
    DOOR.Discharging -> DOOR.Charging_for_Atrium : after(delayVENT_PULSEWIDTH, msec)
    DOOR.Discharging_to_Atrium -> DOOR.Charging : after(delayATR_PULSEWIDTH, msec)
    DOOR.Charging -> DOOR.Discharging : after(delayAV_DELAY, msec)
  AOOR.Charging -> ModeSelect [order 2] : [MODE ~= 4]
  VOOR.Charging -> ModeSelect [order 2] : [MODE ~= 5]
  AAIR.Charging -> ModeSelect [order 2] : [MODE ~= 6]
  VVIR.Charging -> ModeSelect [order 2] : [MODE ~= 7]
  DOO.Charging_for_Atrium -> ModeSelect [order 2] : [MODE ~= 8]
  ModeSelect -> AOO.Charging [order 1] : [MODE == 0]
  ModeSelect -> VOO.Charging [order 2] : [MODE == 1]
  ModeSelect -> DOOR.Charging_for_Atrium [order 10] : [MODE == 9]
  ModeSelect -> DOO.Charging_for_Atrium [order 9] : [MODE == 8]
  ModeSelect -> VVIR.Charging [order 8] : [MODE == 7]
  ModeSelect -> AAIR.Charging [order 7] : [MODE == 6]
  ModeSelect -> VOOR.Charging [order 6] : [MODE == 5]
  ModeSelect -> AAI.Charging [order 3] : [MODE == 2]
  ModeSelect -> VVI.Charging [order 4] : [MODE == 3]
  DOOR.Charging_for_Atrium -> ModeSelect [order 2] : [MODE ~= 9]
  ModeSelect -> AOOR.Charging [order 5] : [MODE == 4]
  VOO.Charging -> ModeSelect [order 2] : [MODE ~= 1]
  AAI.Charging -> ModeSelect [order 2] : [MODE ~= 2]
  VVI.Charging -> ModeSelect [order 2] : [MODE ~= 3]
  (default) -> ModeSelect : {delayINTERVAL = INTERVAL/2,
      |  delayAV_DELAY = AV_DELAY/2,
      |  delayARP = ARP/2,
      |  delayVRP = VRP/2,
      |  delayATR_PULSEWIDTH = ATR_PULSEWIDTH/2,
      |  delayVENT_PULSEWIDTH = VENT_PULSEWIDTH/2}
  AOO.Charging -> ModeSelect [order 2] : [MODE ~= 0]
  data: ATR_GND_CTRL output; VENT_GND_CTRL output; VENT_PACE_CTRL output; Z_ATR_CTRL output; Z_VENT_CTRL output; PACE_GND_CTRL output; PACE_CHARGE_CTRL output; PACING_REF_PWM output; ATR_PACE_CTRL output; INTERVAL input; HIGH local boolean =true; LOW local boolean =false; MODE input uint8; ATR_CMP_REF_PWM output; FRONTEND_CTRL output; VENT_CMP_REF_PWM output; ATR_CMP_DETECT input; VENT_CMP_DETECT input; ARP input uint16; VRP input uint16; ATR_AMPLITUDE input uint8; VENT_AMPLITUDE input uint8; ATR_PULSEWIDTH input uint8; VENT_PULSEWIDTH input uint8; VENT_CMP_THRESH_PWM input uint8; ATR_CMP_THRESH_PWM input uint8; AV_DELAY input uint16; ADAPTED_RATE input; delayVRP local; delayARP local; delayATR_PULSEWIDTH local; delayAV_DELAY local; delayINTERVAL local; delayVENT_PULSEWIDTH local
